simulink model "acc_sim"  (R2022b)
settings: Solver=ode4  StartTime=0.0  StopTime=Tf  FixedStep=Tc  RelTol=1e-3
values from neighbouring files (symbols this model uses):
  Kd = 1    [paraset.m]
  Ki = 2    [paraset.m]
  Kp = 10    [paraset.m]
  tau = 0.5    [paraset.m]
  Vx_d = 30    [paraset.m]
  Vx_i = 15    [paraset.m]
  Vx_th = 60/3.6    (= 16.6666666667)    [paraset.m]
settings Model: Creator=user  LastModifiedBy=user
settings DataIOCC: ReturnWorkspaceOutputs=off

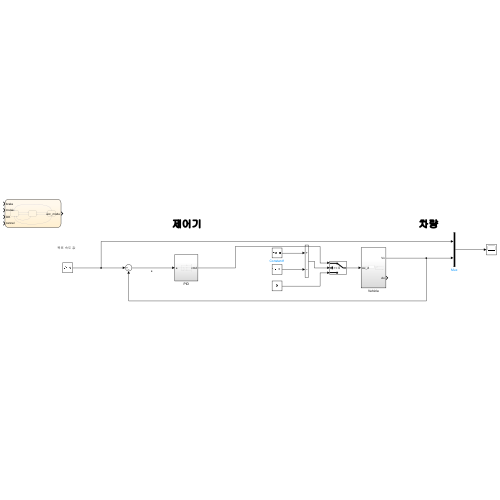
[thumbnail: Simulink's stored preview of the top-level diagram]
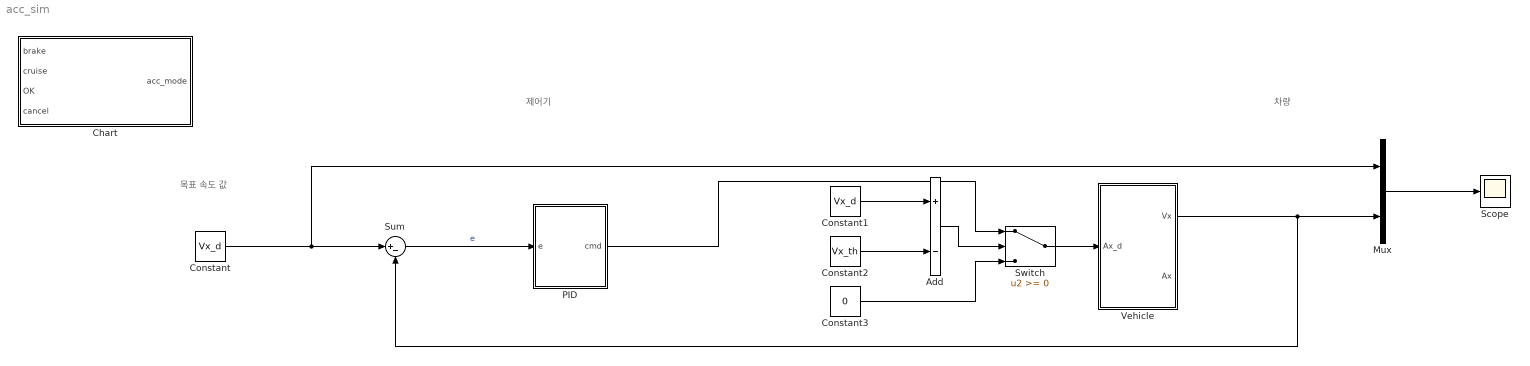
== system acc_sim ==
  note: 목표 속도 값
  note: 차량
  note: 제어기
  Add : Sum  Inputs=+-
  Chart : Stateflow chart  TreatAsAtomicUnit=on
  Constant : Constant  Value=Vx_d
  Constant1 : Constant  Value=Vx_d
  Constant2 : Constant  Value=Vx_th
  Constant3 : Constant  Value=0
  Mux : Mux  Inputs=2
  PID : Subsystem
  Scope : Scope
  Sum : Sum  Inputs=|+-
  Switch : Switch  SaturateOnIntegerOverflow=off  InputSameDT=off
  Vehicle : Subsystem
  wires:
  Sum/1 -> PID/1(e)  "e"
  Vehicle/1(Vx) -> Sum/2, Mux/2
  Mux/1 -> Scope/1
  Constant/1 -> Mux/1, Sum/1
  Switch/1 -> Vehicle/1(Ax_d)
  Constant2/1 -> Add/2
  Constant1/1 -> Add/1
  Add/1 -> Switch/2
  Constant3/1 -> Switch/3
  PID/1(cmd) -> Switch/1

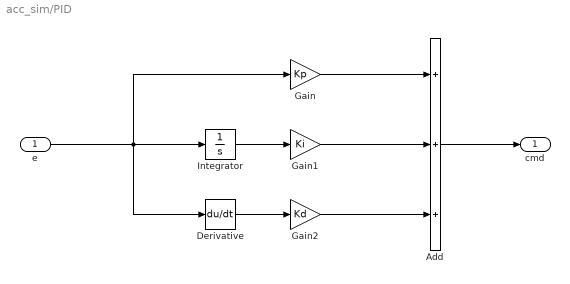
== system acc_sim/PID ==
  e : Inport
  Add : Sum  Inputs=+++
  Derivative : Derivative
  Gain : Gain  Gain=Kp
  Gain1 : Gain  Gain=Ki
  Gain2 : Gain  Gain=Kd
  Integrator : Integrator
  cmd : Outport
  wires:
  Add/1 -> cmd/1
  e/1 -> Derivative/1, Integrator/1, Gain/1
  Gain/1 -> Add/1
  Gain1/1 -> Add/2
  Integrator/1 -> Gain1/1
  Derivative/1 -> Gain2/1
  Gain2/1 -> Add/3

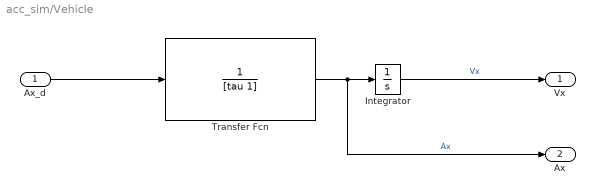
== system acc_sim/Vehicle ==
  Ax_d : Inport
  Integrator : Integrator  InitialCondition=Vx_i
  Transfer Fcn : TransferFcn  Denominator=[tau 1]
  Vx : Outport
  Ax : Outport  Port=2
  wires:
  Transfer Fcn/1 -> Ax/1, Integrator/1  "Ax"
  Ax_d/1 -> Transfer Fcn/1
  Integrator/1 -> Vx/1  "Vx"

== stateflow chart acc_sim/Chart ==
  state ACC_off
    acc_mode = 0;
  state ACC_standby
    acc_mode = 1;
  state ACC_active
    acc_mode = 2;
  ACC_active -> ACC_off [order 3] : [cruise == 0]
  (default) -> ACC_off
  ACC_off -> ACC_standby : [cruise == 1]
  ACC_standby -> ACC_active [order 1] : [OK == 1]
  ACC_active -> ACC_standby [order 1] : [cancel == 1]
  ACC_standby -> ACC_off [order 2] : [cruise == 0]
  ACC_active -> ACC_off [order 2] : [brake == 1]
  ACC_standby -> ACC_off [order 3] : [brake == 1]
  data: brake input; cruise input; OK input; cancel input; acc_mode output
